simulink library "SignalPreprocessingLib"  (R2020b)
settings: Solver=VariableStepAuto  StartTime=0.0  StopTime=10.0  RelTol=1e-3
undefined symbols (not defined in the file or in its folder): fdesignblkfcn, fs, gcbh, param_ecg_gain_mv
(part 6 of 7)

== system SignalPreprocessingLib/Generic Gain + Filtfilter/Enabled Sig Preprocessing Subsystem/Filtfiltering/Bandpass Filter 2 ==
  In : Inport
  Generated Filter Block : DiscreteFir  Tag=BlockMethodSubSystem  Coefficients=[-0.0114243088354877773 0.00587624110456374388 0.00413946068324517157 0.00264334557424035672 0.00138774422276622192 0.00039597756815762733 -0.000357391963790950132 -0.000870027328167087902 -0.00118474210009046274 -0.0013114772414377189 -0.00130211118137258525 -0.00117028348293094116 -0.000969555288066135598 -0.000709991739662891794 -0.000441672338585462343 -0.000165596169411169614 7.38618239838010476e-05 0.000289182992126718261 0.00043918297873611449 0.000554539538172022298 0.000596791094711021305 0.000591852861038305242 0.000558642096174625374 0.000449318410474004379 0.000334719809825502479 0.00020575650819831294 5.39363215079843861e-05 -0.000101322531501510382 -0.000240833690149395291 -0.000354646039305753225 -0.000451018706232981029 -0.000523127741752206499 -0.000570171746042747937 -0.000579976289078059509 -0.000560050610609794802 -0.000510203484091005868 -0.000444253999700439106 -0.000361620699264023418 -0.000270418439597897714 -0.000171285996548194847 -6.96491449474114649e-05 2.51074882581126674e-05 0.000107701466472475207 0.000177443554931332875 0.000215288445749358542 0.000245848468855064048 0.000245696970898627229 0.000229649686627229205 0.00019096241212286473 0.000142984412950488554 7.04459950623022302e-05 -8.24128026295257998e-06 -9.80593727097200246e-05 -0.000181512369773678683 -0.000268731962362029828 -0.000342263684306691809 -0.000409113387221587271 -0.000453067377901137172 -0.000486836085121275519 -0.000497275928952340546 -0.00049828288783324709 -0.000472232231767717378 -0.00043821960462679492 -0.000378588991066479766 -0.000316844305738618603 -0.000241178452312015845 -0.000166037327502541535 -8.72939132895780845e-05 -1.92312446675550752e-05 4.72061762121969014e-05 9.32922079647201252e-05 0.000128677828260322091 0.000142225646220916352 0.000145392718308013161 0.000124316294889322346 9.22525950362868691e-05 3.91139366419743922e-05 -2.09540055264127723e-05 -9.84817072707550728e-05 -0.000176447200533612 -0.000261969930569216219 -0.000338398170707415388 -0.000413673787246831778 -0.000474956484152477126 -0.000526126847064748229 -0.000557031780194342657 -0.000573463759814568652 -0.000565518328802135789 -0.000545968260267525388 -0.000503292825521842527 -0.000450686144492560767 -0.00038193732270500047 -0.000310533512604118864 -0.000229221000311531989 -0.000153634622944792687 -7.7008709436998668e-05 -1.29951882972875049e-05 4.41972427699440645e-05 7.97744827227258452e-05 0.000101355022460052069 9.88614688825825011e-05 8.13696224336354218e-05 3.98982051577762009e-05 -1.42484593806998378e-05 -8.82654671942838254e-05 -0.000167074457359766074 -0.00025963077237387 -0.000347989994374806391 -0.000439444994547399936 -0.00051811479354047299 -0.000590082617058047473 -0.000641838802120880611 -0.000681503522967578934 -0.000694804478821137508 -0.00069209853970065606 -0.000663795693677639645 -0.000621757222242421206 -0.000557224399686986893 -0.000484587241980041772 -0.000396687438130890677 -0.000308737174406251494 -0.000214743893139471981 -0.00013218336614707546 -5.38482479860227792e-05 3.99111044497961476e-06 4.92154210607297082e-05 6.74354760492514721e-05 6.74472479585495194e-05 4.02217001782036176e-05 -4.06942016077313506e-06 -7.33562872444193381e-05 -0.000154074998390272069 -0.000252782754343081062 -0.000354062465090758047 -0.000462222943123069205 -0.000562271536985421011 -0.000658661832374597689 -0.000735808311790427799 -0.000799943578584080828 -0.000838241882526128551 -0.000857844739487072239 -0.000847533102258754556 -0.000817418121589637975 -0.000760200301916437102 -0.000687422833072246636 -0.000595027809558780832 -0.000496080524377292761 -0.000387710990138089018 -0.000284208196984854847 -0.000182518571703508756 -9.84384035011120345e-05 -2.73607674165961268e-05 1.77508990696524649e-05 4.21653277528823839e-05 3.53040248291924125e-05 5.59921773045889137e-06 -5.46825757556310132e-05 -0.000133739024050423885 -0.000236066993422962002 -0.000348549704079315764 -0.000473403235651745358 -0.000595572390038458938 -0.000716976323207035166 ...(+20655 chars)]  InputProcessing=Columns as channels (frame based)
  Out : Outport  VectorParamsAs1DForOutWhenUnconnected=off
  wires:
  In/1 -> Generated Filter Block/1
  Generated Filter Block/1 -> Out/1

== system SignalPreprocessingLib/Generic Gain + Filtfilter/Enabled Sig Preprocessing Subsystem/To Workspace: Gain + Filtfiltered Sig/Enabled To Workspace Subsystem ==
  note: The subsystem is only enabled when it receives a (non-zero) signal
  In1 : Inport
  Enable : EnablePort
  To Workspace : ToWorkspace  VariableName=out_gain_filfiltered_sig  SaveFormat=Structure  SampleTime=-1
  wires:
  In1/1 -> To Workspace/1

== system SignalPreprocessingLib/SCGxyz Gain + Filtfilter/Enabled SCG Preprocessing Subsystem/Filtfiltering/Bandpass Filter 1 ==
  In : Inport
  Generated Filter Block : DiscreteFir  Tag=BlockMethodSubSystem  Coefficients=[-0.00978480817658220967 0.00796999512757378195 0.00147001916949950507 -0.00206976963634554088 -0.00243890991203639124 -0.000924134149517863001 0.000721734906664772908 0.00129711475091687537 0.000656253913654551951 -0.000505332991406271686 -0.0012801272291147899 -0.00118584056106384888 -0.000396379626042962676 0.000462570629011344568 0.00079523934067100995 0.000413152706797699921 -0.000373518377931415205 -0.00101662167067520059 -0.00109601261216027662 -0.000593906547902721513 0.00013435029468211794 0.000600271945192065227 0.000514574052205835205 -5.24294882560059138e-05 -0.000721006732064664153 -0.00106936812684002851 -0.000885784329198623685 -0.000306368867510058802 0.000299921121108211923 0.00055090300805175213 0.000305129539032457354 -0.000280348626867030323 -0.000834835852168314672 -0.00102988416243328038 -0.000749730060181843442 -0.00018384442768847384 0.000330781953284531652 0.000474456713548894286 0.00018715851511990093 -0.00037570651628371528 -0.000841441599320687434 -0.000980583400496216851 -0.000677521760008558955 -0.000143136714861572342 0.000296905261906841298 0.000427455994318532166 0.00013698321512635404 -0.000377779512805234978 -0.000807928899011485448 -0.000914634913299251437 -0.000653887485439495482 -0.000162386642357020724 0.000270410746944910174 0.000394818020750343026 0.000144292032000806675 -0.000318126126834723073 -0.000730717848545356027 -0.000862982022422141819 -0.0006461832253515002 -0.000197068691395214035 0.000227657437070046339 0.000390339376955589645 0.000202019386221156732 -0.000218262841065524645 -0.000630398467646775583 -0.000802033681634044845 -0.000643386601296857597 -0.000239583998883231527 0.000186056910795609839 0.000403403846243817683 0.000291609858585275487 -8.00732001476186567e-05 -0.000501540638877951057 -0.000730203151559393848 -0.000640276523076700071 -0.00027737553443828801 0.000156493764593411161 0.00043156139543532344 0.000397367103231359312 8.29189622619686553e-05 -0.000340599175797182173 -0.000631305624859686211 -0.000622947681400518255 -0.000317342453511192167 0.000133455335091144057 0.000471287365522237995 0.000526528964862326278 0.000266844016988408261 -0.000160112953992838734 -0.000507941523151940531 -0.000580953412745898053 -0.000334693556591401226 0.000109719501491407223 0.000513360648349098832 0.000657877410860213761 0.000469632889523299087 5.66691264257968493e-05 -0.00035174600552400606 -0.000520266671698473124 -0.000342073082939085209 9.47970697972318443e-05 0.000556210436752066603 0.000795382016377131282 0.000685450046798985143 0.000289752333424098715 -0.000168394924182923401 -0.000424984820321057985 -0.000326854493347916676 8.34347145894279147e-05 0.000590237414229303711 0.000924037851917966133 0.000905501272637524823 0.000546953829290044167 5.01002670594704154e-05 -0.000300380671439964494 -0.00029725255069634499 7.24448185066152141e-05 0.000616892125763008367 0.00104469796439719061 0.0011254010687403752 0.000815941579190399566 0.000293722454277149864 -0.000147131313195571635 -0.000243553418517324018 6.68821353140179397e-05 0.000631331563725699208 0.00114457781901217874 0.00133020230521578835 0.00109202570585933685 0.000561661563459188678 4.12191178191941113e-05 -0.000168825603708367067 6.18472916977904128e-05 0.000623699245113693902 0.00121794150913768183 0.0015200947806226976 0.00136753539574389362 0.000847811546795603659 0.000253069734210485946 -7.61054743145556534e-05 5.94169316983781721e-05 0.000599709927775937484 0.00125856843564240545 0.00167936422330872853 0.00163112458376294235 0.00114116904428636801 0.000486071978403662479 3.87954501406567137e-05 5.99888187065994788e-05 0.000552926215869422081 0.00125934973898075798 0.00179616995776612381 0.00186851973153335919 0.00143595292525184009 0.000740124310155826576 0.000171789154674743978 5.84203269058169574e-05 0.000478305096295934275 0.00121446318353966051 0.00186532763417856444 0.00207320507044359784 0.00171914297636467346 0.0010007500900107956 0.000316849149570202051 5.78099051728010543e-05 ...(+13942 chars)]  InputProcessing=Columns as channels (frame based)
  Out : Outport  VectorParamsAs1DForOutWhenUnconnected=off
  wires:
  Generated Filter Block/1 -> Out/1
  In/1 -> Generated Filter Block/1
